simulink model "sina"  (R2016b)
settings: Solver=ode23tb  StartTime=0.0  StopTime=10  MaxStep=1e-4  RelTol=1e-3
undefined symbols (not defined in the file): DiscIntNeverNeededParam
libraries: powerlib x4, eeHysteresisControl x1, simulink x1
settings Model: Creator=80573  LastModifiedBy=Lenovo

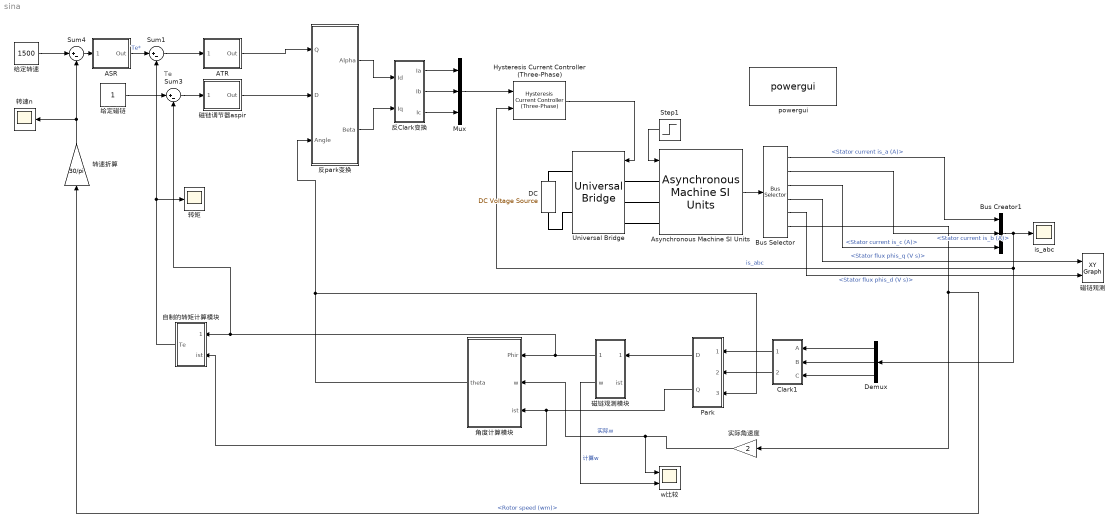
== system sina ==
  note: Te
  ASR : Subsystem  AncestorBlock=|  DialogController=POWERSYS.PowerSysDialog  mask(Discrete PI Controller){Kpw=20, Kiw=0.8, Ba=0, Par_Limits=[30 -30], Init=0, Ts=1.00000000000000e-05}
      | powerlib_extras/Discrete 
      | Control Blocks/Discrete
      | PI Controller
      mask prompts: Kpw "Proportional gain (Kp):"; Kiw "Integral gain (Ki):"; Ba "feedback gain (Ba)"; Par_Limits "Output limits: [ Upper   Lower ]"; Init "Output initial value:"; Ts "Sample time:"
      mask help: This block implements a discrete PI controller.
      mask init:
      | UpperLimit=Par_Limits(1);
      | LowerLimit=Par_Limits(2);
      | power_initmask();
      mask Help: This block is part of a subset of blocks in the Extras library that does not have documentation associated with it, other than the block mask description.
      mask Display: disp('PI');
  ATR : Subsystem  AncestorBlock=|  DialogController=POWERSYS.PowerSysDialog  mask(Discrete PI Controller){Kpw=4.5, Kiw=12, Ba=0, Par_Limits=[60 -60], Init=0, Ts=1.00000000000000e-05}
      | powerlib_extras/Discrete 
      | Control Blocks/Discrete
      | PI Controller
      mask prompts: Kpw "Proportional gain (Kp):"; Kiw "Integral gain (Ki):"; Ba "feedback gain (Ba)"; Par_Limits "Output limits: [ Upper   Lower ]"; Init "Output initial value:"; Ts "Sample time:"
      mask help: This block implements a discrete PI controller.
      mask init:
      | UpperLimit=Par_Limits(1);
      | LowerLimit=Par_Limits(2);
      | power_initmask();
      mask Help: This block is part of a subset of blocks in the Extras library that does not have documentation associated with it, other than the block mask description.
      mask Display: disp('PI');
  Asynchronous Machine SI Units : powerlib/Machines/Asynchronous Machine SI Units  RotorType=Squirrel-cage  PresetModel=No  MechanicalLoad=Torque Tm  ShowDetailedParameters=on  ReferenceFrame=Stationary  Units=SI  MeasurementBus=off  NominalParameters=[7500 380 50]  Stator=[0.7384 0.003045]  Rotor=[0.07402 0.003045]  Cage1=[0.4155 0.002066]  Cage2=[0.4168 0.0003495]  Lm=0.1241  Mechanical=[0.0343 0 2]  PolePairs=2  InitialConditions=[1 0 0 0 0 0 0 0]  SimulateSaturation=off  Saturation=[14.03593122, 27.81365428, 53.79336849, 72.68890987, 97.98006896, 148.6815601, 215.7428561, 302.9841135, 428.7778367 ; 230, 322, 414, 460, 506, 552, 598, 644, 690]  LoadFlowParameters=1492000  TsPowergui=0  TsBlock=-1  IterativeModel=Trapezoidal non iterative  IterativeDiscreteModel=Trapezoidal non iterative  Pmec=1.492e+006
  Bus Creator1 : BusCreator  Inputs=3
  Bus Selector : BusSelector  OutputSignals=Stator measurements.Stator current is_a (A),Stator measurements.Stator current is_b (A),Stator measurements.Stator current is_c (A),Stator measurements.Stator flux phis_q (V s),Stator measurements.Stator flux phis_d (V s),Mechanical.Rotor speed (wm)
  Clark1 : Subsystem
  DC : powerlib/Electrical Sources/DC Voltage Source  Amplitude=510  Measurements=None
  Demux : Demux  Outputs=3
  Hysteresis Current Controller (Three-Phase) : eeHysteresisControl/Hysteresis Current Controller (Three-Phase)  h=1  Ts=-1
  Mux : Mux  Inputs=3
  Park : Subsystem
  Step1 : Step  After=2  SampleTime=0
  Sum1 : Sum  Inputs=|+-
  Sum3 : Sum  Inputs=|+-
  Sum4 : Sum  Inputs=|+-
  Universal Bridge : powerlib/Power Electronics/Universal Bridge  Arms=3  SnubberResistance=1e5  SnubberCapacitance=inf  Device=IGBT / Diodes  Ron=1e-3  Lon=0  ForwardVoltages="[  0  0  ]"  ForwardVoltage=0  GTOparameters=[ 10e-6 , 20e-6 ]  IGBTparameters=[ 1e-6 , 2e-6 ]  Measurements=None  Measurements_2=None  converterType=Rectifier
  is_abc : Scope
  powergui : powerlib/powergui  SimulationMode=Discrete  SampleTime=0.00001  frequency=50  Iterations=50  frequencyindice=50  Pbase=100e6  ErrMax=1e-4  UnitsV=kV  UnitsW=MW  buscounter=0  FunctionMessages=off  echomessages=off  EnableUseOfTLC=off  CurrentSourceSwitches=off  DisableSnubberDevices=off  DisableRonSwitches=off  DisableVfSwitches=off  DisplayEquations=off  AutomaticDiscreteSolvers=off  SolverType=Tustin/Backward Euler (TBE)  Interpol=off  ExternalGateDelay=off  methode=off  Ts=100  x0status=zero  SPID=on  SwTol=0  HookPort=off  NonlinearTolerance=1e-4  nMaxIteration=100  ContinueOnMaxIteration=off  RestoreLinks=warning  ResistiveCurrentMeasurement=off  Frange=[0:2:500]  Ylog=off  Xlog=on  ShowGrid=off  save=off  variable=ZData  structure=0  ZoomFFT=on  StartTime=0.0  cycles=1  DisplayStyle=1  fundamental=60  FreqAxis=off  MaxFrequency=1000  frequencyindicesteady=1  RmsSteady=1  display=off
  w比较 : Scope  NumInputPorts=2
  反Clark变换 : Subsystem
  反park变换 : Subsystem
  实际角速度 : Gain  Gain=2
  磁链观测 : simulink/Sinks/XY Graph  xmin=-1  xmax=1  ymin=-1  ymax=1  st=-1
  磁链观测模块 : Subsystem
  磁链调节器aspir : Subsystem  AncestorBlock=|  DialogController=POWERSYS.PowerSysDialog  mask(Discrete PI Controller){Kpw=1.8, Kiw=100, Ba=0, Par_Limits=[13 -13], Init=0, Ts=1.00000000000000e-05}
      | powerlib_extras/Discrete 
      | Control Blocks/Discrete
      | PI Controller
      mask prompts: Kpw "Proportional gain (Kp):"; Kiw "Integral gain (Ki):"; Ba "feedback gain (Ba)"; Par_Limits "Output limits: [ Upper   Lower ]"; Init "Output initial value:"; Ts "Sample time:"
      mask help: This block implements a discrete PI controller.
      mask init:
      | UpperLimit=Par_Limits(1);
      | LowerLimit=Par_Limits(2);
      | power_initmask();
      mask Help: This block is part of a subset of blocks in the Extras library that does not have documentation associated with it, other than the block mask description.
      mask Display: disp('PI');
  给定磁链 : Constant
  给定转速 : Constant  Value=1500
  自制的转矩计算模块 : Subsystem
  角度计算模块 : Subsystem
  转矩 : Scope
  转速n : Scope
  转速折算 : Gain  Gain=30/pi
  wires:
  Step1/1 -> Asynchronous Machine SI Units/1
  Park/1(D) -> 磁链观测模块/1(ism)
  Park/2(Q) -> 自制的转矩计算模块/2(ist), 角度计算模块/3(ist)
  Sum1/1 -> ATR/1(Error)
  Sum3/1 -> 磁链调节器aspir/1(Error)
  Sum4/1 -> ASR/1(Error)
  给定磁链/1 -> Sum3/1
  Mux/1 -> Hysteresis Current Controller (Three-Phase)/1
  角度计算模块/1(theta) -> 反park变换/3(Angle), Park/3(Angle)
  反Clark变换/1(Ia) -> Mux/1
  Bus Selector/1 -> Bus Creator1/1  "<Stator current is_a (A)>"
  Bus Selector/3 -> Bus Creator1/3  "<Stator current is_c (A)>"
  Bus Selector/4 -> 磁链观测/1  "<Stator flux phis_q (V s)>"
  Bus Selector/5 -> 磁链观测/2  "<Stator flux phis_d (V s)>"
  Bus Selector/2 -> Bus Creator1/2  "<Stator current is_b (A)>"
  Bus Selector/6 -> 转速折算/1, 实际角速度/1  "<Rotor speed (wm)>"
  Bus Creator1/1 -> Demux/1, Hysteresis Current Controller (Three-Phase)/2, is_abc/1  "is_abc"
  Asynchronous Machine SI Units/1 -> Bus Selector/1
  Hysteresis Current Controller (Three-Phase)/1 -> Universal Bridge/1
  实际角速度/1 -> 角度计算模块/2(w), w比较/1  "实际w"
  磁链观测模块/2(w) -> w比较/2  "计算w"
  磁链调节器aspir/1(Out) -> 反park变换/2(D)
  ATR/1(Out) -> 反park变换/1(Q)
  反park变换/1(Alpha) -> 反Clark变换/1(Id)
  反park变换/2(Beta) -> 反Clark变换/2(Iq)
  给定转速/1 -> Sum4/1
  转速折算/1 -> 转速n/1, Sum4/2
  反Clark变换/3(Ic) -> Mux/3
  反Clark变换/2(Ib) -> Mux/2
  ASR/1(Out) -> Sum1/1  "Te*"
  Clark1/1(Alpha) -> Park/1(Alpha)
  Clark1/2(Beta) -> Park/2(Beta)
  Demux/1 -> Clark1/1(A)
  Demux/2 -> Clark1/2(B)
  Demux/3 -> Clark1/3(C)
  磁链观测模块/1(Phir) -> Sum3/2, 自制的转矩计算模块/1(phir), 角度计算模块/1(Phir)
  自制的转矩计算模块/1(Te) -> 转矩/1, Sum1/2
  connections:
  Universal Bridge/LConn1 -- Asynchronous Machine SI Units/LConn1
  Universal Bridge/LConn3 -- Asynchronous Machine SI Units/LConn3
  DC/LConn1 -- Universal Bridge/RConn2
  Universal Bridge/LConn2 -- Asynchronous Machine SI Units/LConn2
  DC/RConn1 -- Universal Bridge/RConn1

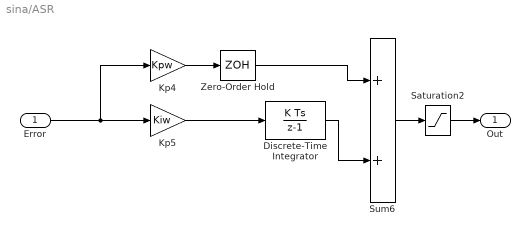
== system sina/ASR ==
  Error : Inport  SampleTime=Ts
  Discrete-Time Integrator : DiscreteIntegrator  InitialCondition=Init  SampleTime=Ts  OutMin=[-80]  OutMax=[80]  LimitOutput=on  UpperSaturationLimit=UpperLimit  LowerSaturationLimit=LowerLimit  ICPrevOutput=DiscIntNeverNeededParam  ICPrevScaledInput=DiscIntNeverNeededParam
  Kp4 : Gain  Gain=Kpw  SaturateOnIntegerOverflow=on  SampleTime=Ts  OutDataTypeStr=Inherit: Same as input  ParamDataTypeStr=Inherit: Same as input
  Kp5 : Gain  Gain=Kiw  SaturateOnIntegerOverflow=on  SampleTime=Ts  OutDataTypeStr=Inherit: Same as input  ParamDataTypeStr=Inherit: Same as input
  Saturation2 : Saturate  UpperLimit=UpperLimit  LowerLimit=LowerLimit  SampleTime=Ts  OutMin=[-75]  OutMax=[75]
  Sum6 : Sum  InputSameDT=on  SaturateOnIntegerOverflow=on  SampleTime=Ts  OutDataTypeStr=Inherit: Same as first input
  Zero-Order Hold : ZeroOrderHold  SampleTime=Ts
  Out : Outport  SampleTime=Ts  InitialOutput=0
  wires:
  Error/1 -> Kp5/1, Kp4/1
  Zero-Order Hold/1 -> Sum6/1
  Saturation2/1 -> Out/1
  Discrete-Time Integrator/1 -> Sum6/2
  Kp4/1 -> Zero-Order Hold/1
  Kp5/1 -> Discrete-Time Integrator/1
  Sum6/1 -> Saturation2/1

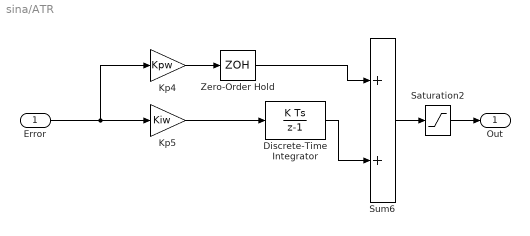
== system sina/ATR ==
  Error : Inport  SampleTime=Ts
  Discrete-Time Integrator : DiscreteIntegrator  InitialCondition=Init  SampleTime=Ts  OutMin=[-65]  OutMax=[65]  LimitOutput=on  UpperSaturationLimit=UpperLimit  LowerSaturationLimit=LowerLimit  ICPrevOutput=DiscIntNeverNeededParam  ICPrevScaledInput=DiscIntNeverNeededParam
  Kp4 : Gain  Gain=Kpw  SaturateOnIntegerOverflow=on  SampleTime=Ts  OutDataTypeStr=Inherit: Same as input  ParamDataTypeStr=Inherit: Same as input
  Kp5 : Gain  Gain=Kiw  SaturateOnIntegerOverflow=on  SampleTime=Ts  OutDataTypeStr=Inherit: Same as input  ParamDataTypeStr=Inherit: Same as input
  Saturation2 : Saturate  UpperLimit=UpperLimit  LowerLimit=LowerLimit  SampleTime=Ts  OutMin=[-60]  OutMax=[60]
  Sum6 : Sum  InputSameDT=on  SaturateOnIntegerOverflow=on  SampleTime=Ts  OutDataTypeStr=Inherit: Same as first input
  Zero-Order Hold : ZeroOrderHold  SampleTime=Ts
  Out : Outport  SampleTime=Ts  InitialOutput=0
  wires:
  Error/1 -> Kp5/1, Kp4/1
  Zero-Order Hold/1 -> Sum6/1
  Saturation2/1 -> Out/1
  Discrete-Time Integrator/1 -> Sum6/2
  Kp4/1 -> Zero-Order Hold/1
  Kp5/1 -> Discrete-Time Integrator/1
  Sum6/1 -> Saturation2/1

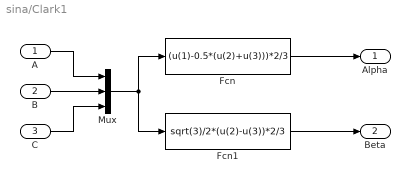
== system sina/Clark1 ==
  A : Inport
  B : Inport  Port=2
  C : Inport  Port=3
  Fcn : Fcn  Expr=(u(1)-0.5*(u(2)+u(3)))*2/3
  Fcn1 : Fcn  Expr=sqrt(3)/2*(u(2)-u(3))*2/3
  Mux : Mux  Inputs=3
  Alpha : Outport
  Beta : Outport  Port=2
  wires:
  B/1 -> Mux/2
  Mux/1 -> Fcn1/1, Fcn/1
  Fcn1/1 -> Beta/1
  Fcn/1 -> Alpha/1
  C/1 -> Mux/3
  A/1 -> Mux/1

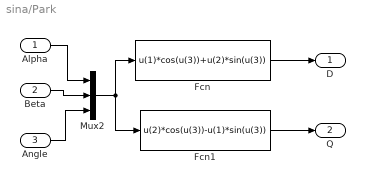
== system sina/Park ==
  Alpha : Inport
  Beta : Inport  Port=2
  Angle : Inport  Port=3
  Fcn : Fcn  Expr=u(1)*cos(u(3))+u(2)*sin(u(3))
  Fcn1 : Fcn  Expr=u(2)*cos(u(3))-u(1)*sin(u(3))
  Mux2 : Mux  Inputs=3
  D : Outport
  Q : Outport  Port=2
  wires:
  Beta/1 -> Mux2/2
  Mux2/1 -> Fcn1/1, Fcn/1
  Angle/1 -> Mux2/3
  Alpha/1 -> Mux2/1
  Fcn1/1 -> Q/1
  Fcn/1 -> D/1

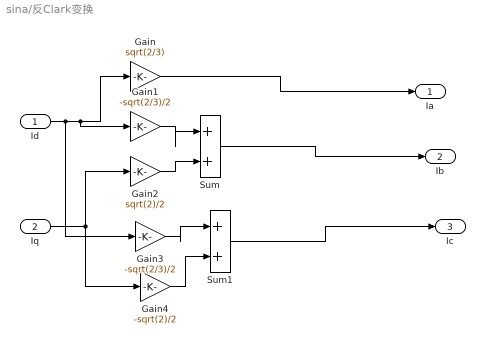
== system sina/反Clark变换 ==
  Id : Inport
  Iq : Inport  Port=2
  Gain : Gain  Gain=sqrt(2/3)  SaturateOnIntegerOverflow=on  OutDataTypeStr=Inherit: Same as input  ParamDataTypeStr=Inherit: Same as input
  Gain1 : Gain  Gain=-sqrt(2/3)/2  SaturateOnIntegerOverflow=on  OutDataTypeStr=Inherit: Same as input  ParamDataTypeStr=Inherit: Same as input
  Gain2 : Gain  Gain=sqrt(2)/2  SaturateOnIntegerOverflow=on  OutDataTypeStr=Inherit: Same as input  ParamDataTypeStr=Inherit: Same as input
  Gain3 : Gain  Gain=-sqrt(2/3)/2  SaturateOnIntegerOverflow=on  OutDataTypeStr=Inherit: Same as input  ParamDataTypeStr=Inherit: Same as input
  Gain4 : Gain  Gain=-sqrt(2)/2  SaturateOnIntegerOverflow=on  OutDataTypeStr=Inherit: Same as input  ParamDataTypeStr=Inherit: Same as input
  Sum : Sum  Inputs=|++  SaturateOnIntegerOverflow=on
  Sum1 : Sum  Inputs=|++  SaturateOnIntegerOverflow=on
  Ia : Outport
  Ib : Outport  Port=2
  Ic : Outport  Port=3
  wires:
  Id/1 -> Gain/1, Gain1/1, Gain3/1
  Gain/1 -> Ia/1
  Iq/1 -> Gain2/1, Gain4/1
  Gain1/1 -> Sum/1
  Gain2/1 -> Sum/2
  Sum/1 -> Ib/1
  Gain3/1 -> Sum1/1
  Gain4/1 -> Sum1/2
  Sum1/1 -> Ic/1

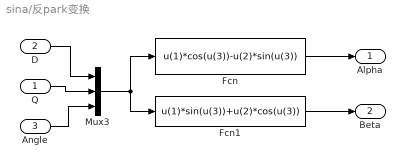
== system sina/反park变换 ==
  Q : Inport
  D : Inport  Port=2
  Angle : Inport  Port=3
  Fcn : Fcn  Expr=u(1)*cos(u(3))-u(2)*sin(u(3))
  Fcn1 : Fcn  Expr=u(1)*sin(u(3))+u(2)*cos(u(3))
  Mux3 : Mux  Inputs=3
  Alpha : Outport
  Beta : Outport  Port=2
  wires:
  Angle/1 -> Mux3/3
  Fcn1/1 -> Beta/1
  Mux3/1 -> Fcn1/1, Fcn/1
  Fcn/1 -> Alpha/1
  D/1 -> Mux3/1
  Q/1 -> Mux3/2

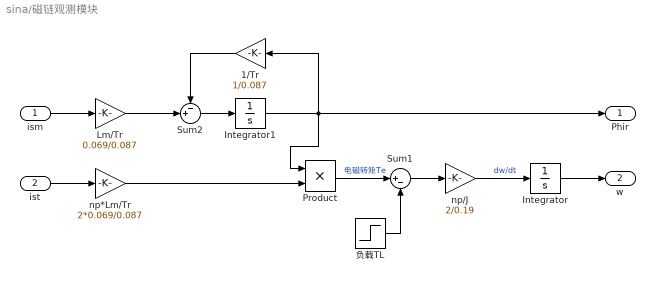
== system sina/磁链观测模块 ==
  ism : Inport
  ist : Inport  Port=2
  1/Tr : Gain  Gain=1/0.087
  Integrator : Integrator
  Integrator1 : Integrator  InitialCondition=1e-5
  Lm/Tr : Gain  Gain=0.069/0.087
  Product : Product
  Sum1 : Sum  Inputs=|+-
  Sum2 : Sum  Inputs=-+|
  np*Lm/Tr : Gain  Gain=2*0.069/0.087
  np/J : Gain  Gain=2/0.19
  负载TL : Step  Time=0.6  After=55  SampleTime=0
  Phir : Outport
  w : Outport  Port=2
  wires:
  Sum2/1 -> Integrator1/1
  Integrator1/1 -> Phir/1, Product/1, 1/Tr/1
  Sum1/1 -> np/J/1
  np*Lm/Tr/1 -> Product/2
  ism/1 -> Lm/Tr/1
  Lm/Tr/1 -> Sum2/2
  ist/1 -> np*Lm/Tr/1
  Integrator/1 -> w/1
  负载TL/1 -> Sum1/2
  np/J/1 -> Integrator/1  "dw/dt"
  Product/1 -> Sum1/1  "电磁转矩Te"
  1/Tr/1 -> Sum2/1

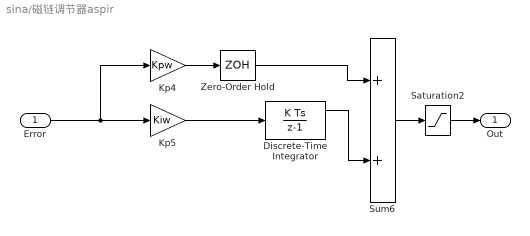
== system sina/磁链调节器aspir ==
  Error : Inport  SampleTime=Ts
  Discrete-Time Integrator : DiscreteIntegrator  InitialCondition=Init  SampleTime=Ts  OutMin=[-15]  OutMax=[15]  LimitOutput=on  UpperSaturationLimit=UpperLimit  LowerSaturationLimit=LowerLimit  ShowSaturationPort=on  ShowStatePort=on  ICPrevOutput=DiscIntNeverNeededParam  ICPrevScaledInput=DiscIntNeverNeededParam
  Kp4 : Gain  Gain=Kpw  SaturateOnIntegerOverflow=on  SampleTime=Ts  OutDataTypeStr=Inherit: Same as input  ParamDataTypeStr=Inherit: Same as input
  Kp5 : Gain  Gain=Kiw  SaturateOnIntegerOverflow=on  SampleTime=Ts  OutDataTypeStr=Inherit: Same as input  ParamDataTypeStr=Inherit: Same as input
  Saturation2 : Saturate  UpperLimit=UpperLimit  LowerLimit=LowerLimit  SampleTime=Ts  OutMin=[-15]  OutMax=[15]
  Sum6 : Sum  InputSameDT=on  SaturateOnIntegerOverflow=on  SampleTime=Ts  OutDataTypeStr=Inherit: Same as first input
  Zero-Order Hold : ZeroOrderHold  SampleTime=Ts
  Out : Outport  SampleTime=Ts  InitialOutput=0
  wires:
  Error/1 -> Kp5/1, Kp4/1
  Zero-Order Hold/1 -> Sum6/1
  Saturation2/1 -> Out/1
  Discrete-Time Integrator/1 -> Sum6/2
  Kp4/1 -> Zero-Order Hold/1
  Kp5/1 -> Discrete-Time Integrator/1
  Sum6/1 -> Saturation2/1

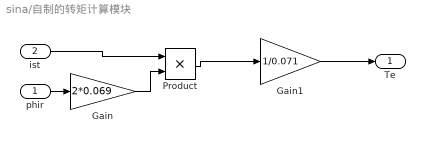
== system sina/自制的转矩计算模块 ==
  phir : Inport
  ist : Inport  Port=2
  Gain : Gain  Gain=2*0.069
  Gain1 : Gain  Gain=1/0.071
  Product : Product
  Te : Outport
  wires:
  ist/1 -> Product/1
  Gain/1 -> Product/2
  Gain1/1 -> Te/1
  Product/1 -> Gain1/1
  phir/1 -> Gain/1

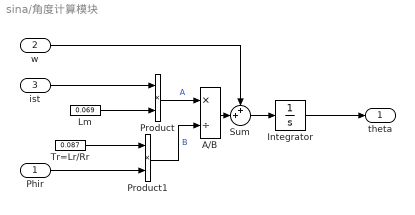
== system sina/角度计算模块 ==
  Phir : Inport
  w : Inport  Port=2
  ist : Inport  Port=3
  A/B : Product  Inputs=*/
  Integrator : Integrator
  Lm : Constant  Value=0.069
  Product : Product
  Product1 : Product
  Sum : Sum  Inputs=++|
  Tr=Lr/Rr : Constant  Value=0.087
  theta : Outport
  wires:
  ist/1 -> Product/1
  w/1 -> Sum/1
  Product/1 -> A/B/1  "A"
  Sum/1 -> Integrator/1
  Integrator/1 -> theta/1
  Product1/1 -> A/B/2  "B"
  Lm/1 -> Product/2
  A/B/1 -> Sum/2
  Phir/1 -> Product1/2
  Tr=Lr/Rr/1 -> Product1/1
